simulink model "vanderpol"  (R2022b)
settings: Solver=ode5  StartTime=0.0  StopTime=7  FixedStep=0.01  RelTol=1e-3
settings Model: Creator=b6062805  LastModifiedBy=b6062805
settings DataIOCC: SaveFormat=Structure  SignalLogging=off  DSMLogging=off  ReturnWorkspaceOutputs=off

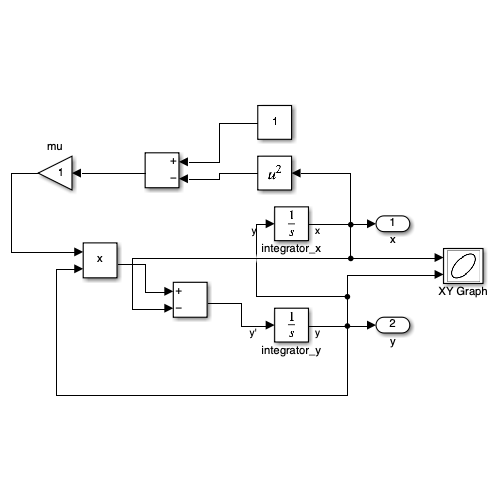
[thumbnail: Simulink's stored preview of the top-level diagram]
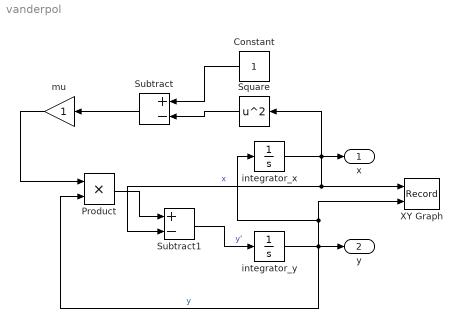
== system vanderpol ==
  Constant : Constant
  Product : Product
  Square : Math  Operator=square
  Subtract : Sum  Inputs=+-
  Subtract1 : Sum  Inputs=+-
  XY Graph : Record  FileSettingsInternal="{\"entries\":[{\"content\":{\"excelSettings\":{\"content\":{},\"type\":\"Streamout.ExcelSettings\"}},\"type\":\"Streamout.FileSettingStorage\",\"uuid\":\"ea26d9f8-25b3-404c-aca2-06e25c069784\"}],\"packageUris\":[\"http://schema.mathworks.com/mf0/streamout_blocks/R2020a\"],\"version\":\"1.0\"}"  Layout=[1 1]  SignalsInternal="{\"entries\":[{\"content\":{\"signals\":[{\"content\":{\"blockPath\":[\"vanderpol/XY Graph\"],\"channel\":[],\"dimensions\":[1],\"domain\":\"vanderpol/XY Graph\",\"lineColor\":\"#a2142f\",\"plots\":[1],\"port\":1,\"sid\":[\"\"],\"signalID\":5595,\"signalName\":\"x\"},\"type\":\"RecordBlkView.Signal\",\"uuid\":\"51479424-79bc-4470-813b-d9971b4bc8b0\"},{\"content\":{\"blockPath\":[\"vanderpol/XY Graph\"],\"channel\":[],\"dimensions\":[1],\"domain\":\"vanderpol/XY Graph\",\"lineColor\":\"#139fff\",\"plots\":[1],\"port\":2,\"sid\":[\"\"],\"signalID\":5599,\"signalName\":\"y\"},\"type\":\"RecordBlkView.Signal\",\"uuid\":\"7f2ea63e-59c0-4daf-a18a-500aacd4c222\"}]},\"type\":\"RecordBlkView.InputSignals\",\"uuid\":\"fefa0657-324e-4bbc-9701-cd9839a864da\"}],\"packageUris\":[\"http://schema.mathworks.com/mf0/streamout_blocks/R2020a\"],\"version\":\"1.0\"}"  VisualizationBindings="{\"xyplotplugin\":{\"info\":[{\"series\":[{\"bindingParametersList\":[{\"parameter\":\"X-Axis\",\"signalID\":5595,\"signalName\":\"x\"},{\"parameter\":\"Y-Axis\",\"signalID\":5599,\"signalName\":\"y\"}],\"seriesID\":53039}],\"subplotID\":1}]}}"  CompatibilityTag=XY
  integrator_x : Integrator  InitialCondition=1.25
  integrator_y : Integrator  InitialCondition=2.25
  mu : Gain
  x : Outport
  y : Outport  Port=2
  wires:
  integrator_x/1 -> XY Graph/1, Subtract1/2, x/1, Square/1  "x"
  integrator_y/1 -> y/1, XY Graph/2, integrator_x/1, Product/2  "y"
  Square/1 -> Subtract/2
  Constant/1 -> Subtract/1
  Subtract/1 -> mu/1
  mu/1 -> Product/1
  Product/1 -> Subtract1/1
  Subtract1/1 -> integrator_y/1  "y'"
